simulink model "Posture_Regulation_NO_Singularity"  (R2022b)
settings: Solver=FixedStepAuto  StartTime=0.0  StopTime=10.0  MaxStep=0.1  RelTol=1e-3
values from neighbouring files (symbols this model uses):
  K = [3, 3, 1]    [AutomatedSimulation.m]
  theta_f = deg2rad(fc(3))    [AutomatedSimulation.m]
  theta_i = deg2rad(ans.output.signals.values(end,3))    [AutomatedSimulation.m]
  x_f = fc(1)    [AutomatedSimulation.m]
  x_i = ans.output.signals.values(end,1)    [AutomatedSimulation.m]
  y_f = fc(2)    [AutomatedSimulation.m]
  y_i = ans.output.signals.values(end,2)    [AutomatedSimulation.m]
libraries: simulink_extras x2
settings Model: Creator=Musta  LastModifiedBy=Musta

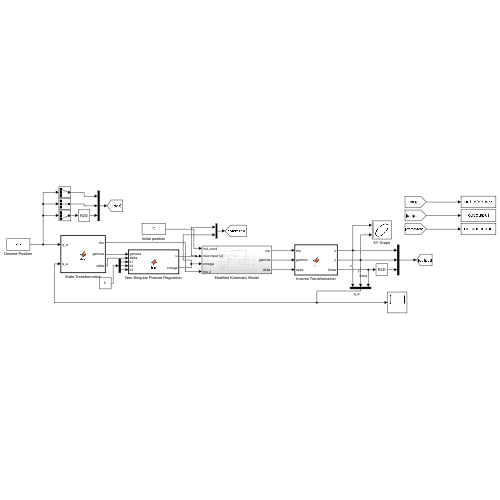
[thumbnail: Simulink's stored preview of the top-level diagram]
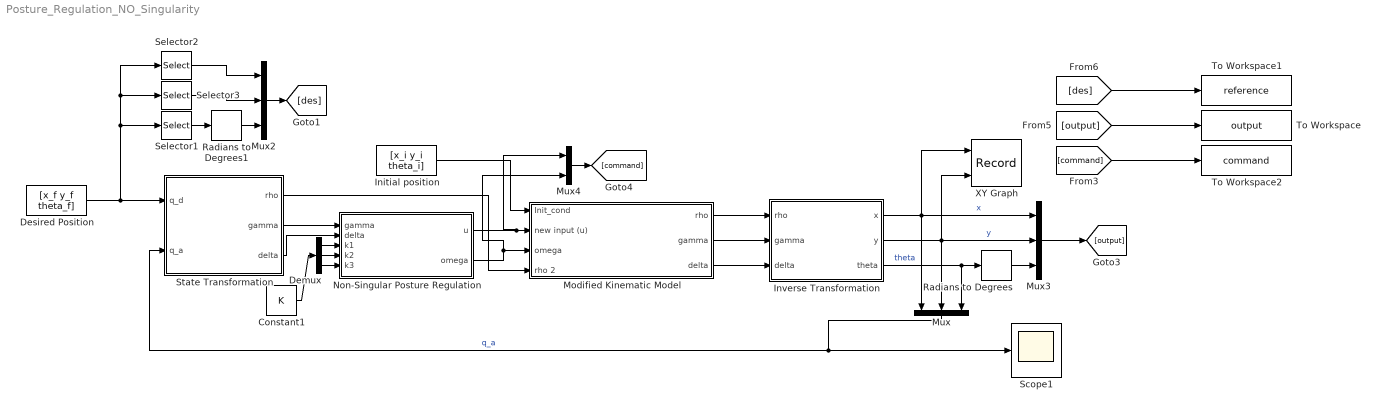
== system Posture_Regulation_NO_Singularity ==
  Constant1 : Constant  Value=K
  Demux : Demux  Outputs=3
  Desired Position : Constant  Value=[x_f y_f theta_f]
  Initial position : Constant  Value=[x_i y_i theta_i]
  Inverse Transformation : MATLAB Function  TreatAsAtomicUnit=on
  Modified Kinematic Model : Subsystem
  Mux : Mux  Inputs=3
  Mux2 : Mux  Inputs=3
  Mux3 : Mux  Inputs=3
  Mux4 : Mux  Inputs=2
  Non-Singular Posture Regulation : MATLAB Function  TreatAsAtomicUnit=on
  Radians to Degrees : simulink_extras/Transformations/Radians to Degrees
  Radians to Degrees1 : simulink_extras/Transformations/Radians to Degrees
  Scope1 : Scope
  Selector1 : Selector  InputPortWidth=3  IndexOptions=Index vector (dialog)  Indices=3  OutputSizes=1
  Selector2 : Selector  InputPortWidth=3  IndexOptions=Index vector (dialog)  Indices=1  OutputSizes=1
  Selector3 : Selector  InputPortWidth=3  IndexOptions=Index vector (dialog)  Indices=2  OutputSizes=1
  State Transformation : MATLAB Function  TreatAsAtomicUnit=on
  To Workspace : ToWorkspace  VariableName=output  SaveFormat=Structure With Time  SampleTime=-1
  To Workspace1 : ToWorkspace  VariableName=reference  SaveFormat=Structure With Time  SampleTime=-1
  To Workspace2 : ToWorkspace  VariableName=command  SaveFormat=Structure With Time  SampleTime=-1
  XY Graph : Record  FileSettingsInternal="{\"entries\":[{\"content\":{\"excelSettings\":{\"content\":{},\"type\":\"Streamout.ExcelSettings\"}},\"type\":\"Streamout.FileSettingStorage\",\"uuid\":\"c30e0c7c-8de7-4fd5-93f6-f23722b5ae44\"}],\"packageUris\":[\"http://schema.mathworks.com/mf0/streamout_blocks/R2020a\"],\"version\":\"1.0\"}"  Layout=[1 1]  SignalsInternal="{\"entries\":[{\"content\":{\"signals\":[{\"content\":{\"blockPath\":[\"Posture_Regulation_NO_Singularity/XY Graph\"],\"channel\":[],\"dimensions\":[1],\"domain\":\"Posture_Regulation_NO_Singularity/XY Graph\",\"lineColor\":\"#77ac30\",\"plots\":[],\"port\":1,\"sid\":[],\"signalID\":354,\"signalName\":\"x\"},\"type\":\"RecordBlkView.Signal\",\"uuid\":\"1f9c0edf-91b7-4929-98cb-a57c689434ed\"},{\"content\":{\"blockPath\":[\"Posture_Regulation_NO_Singularity/XY Graph\"],\"channel\":[],\"dimensions\":[1],\"domain\":\"Posture_Regulation_NO_Singularity/XY Graph\",\"lineColor\":\"#4dbeee\",\"plots\":[],\"port\":2,\"sid\":[],\"signalID\":357,\"signalName\":\"y\"},\"type\":\"RecordBlkView.Signal\",\"uuid\":\"3df65c5c-25b3-4ef8-84f3-e62cc3054bc7\"}]},\"type\":\"RecordBlkView.InputSignals\",\"uuid\":\"319c4578-7599-4632-be24-bc243958fcb7\"}],\"packageUris\":[\"http://schema.mathworks.com/mf0/streamout_blocks/R2020a\"],\"version\":\"1.0\"}"  VisualizationBindings="{\"xyplotplugin\":{\"info\":[{\"series\":[],\"subplotID\":1}]}}"  CompatibilityTag=XY
  wires:
  [command] -> To Workspace2/1
  [des] -> To Workspace1/1
  [output] -> To Workspace/1
  Selector2/1 -> Mux2/1
  Mux/1 -> Scope1/1, State Transformation/2(q_a)  "q_a"
  Selector3/1 -> Mux2/2
  Inverse Transformation/1(x) -> XY Graph/1, Mux/1, Mux3/1  "x"
  Desired Position/1 -> Selector2/1, Selector3/1, Selector1/1, State Transformation/1(q_d)
  Inverse Transformation/3(theta) -> Mux/3, Radians to Degrees/1  "theta"
  Radians to Degrees/1 -> Mux3/3
  Inverse Transformation/2(y) -> XY Graph/2, Mux3/2, Mux/2  "y"
  Modified Kinematic Model/3(delta) -> Inverse Transformation/3(delta)
  Mux2/1 -> [des]
  State Transformation/1(rho) -> Modified Kinematic Model/4(rho 2)
  Radians to Degrees1/1 -> Mux2/3
  Selector1/1 -> Radians to Degrees1/1
  Modified Kinematic Model/1(rho) -> Inverse Transformation/1(rho)
  Mux4/1 -> [command]
  State Transformation/2(gamma) -> Non-Singular Posture Regulation/1(gamma)
  Modified Kinematic Model/2(gamma) -> Inverse Transformation/2(gamma)
  State Transformation/3(delta) -> Non-Singular Posture Regulation/2(delta)
  Initial position/1 -> Modified Kinematic Model/1(Init_cond)
  Non-Singular Posture Regulation/1(u) -> Mux4/1, Modified Kinematic Model/2(new input (u))
  Mux3/1 -> [output]
  Non-Singular Posture Regulation/2(omega) -> Mux4/2, Modified Kinematic Model/3(omega)
  Constant1/1 -> Demux/1
  Demux/1 -> Non-Singular Posture Regulation/3(k1)
  Demux/2 -> Non-Singular Posture Regulation/4(k2)
  Demux/3 -> Non-Singular Posture Regulation/5(k3)

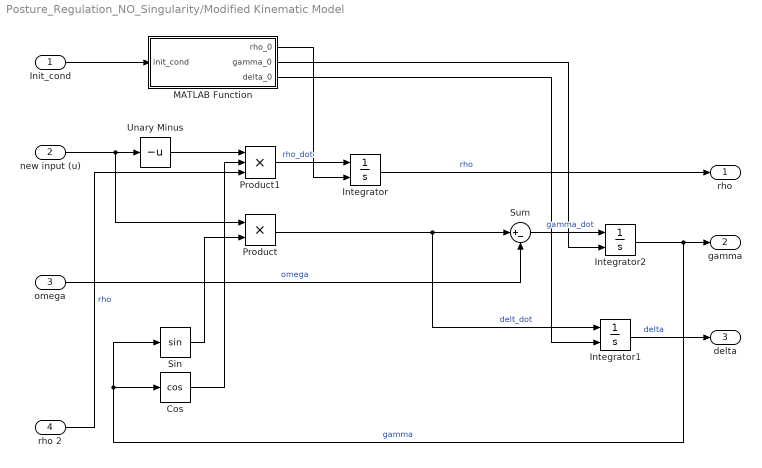
== system Posture_Regulation_NO_Singularity/Modified Kinematic Model ==
  Init_cond : Inport
  new input (u) : Inport  Port=2
  omega : Inport  Port=3
  rho 2 : Inport  Port=4
  Cos : Trigonometry  Operator=cos
  Integrator : Integrator  InitialConditionSource=external  InitialCondition=-10
  Integrator1 : Integrator  InitialConditionSource=external
  Integrator2 : Integrator  InitialConditionSource=external
  MATLAB Function : MATLAB Function  TreatAsAtomicUnit=on
  Product : Product
  Product1 : Product  Inputs=3
  Sin : Trigonometry
  Sum : Sum  Inputs=|+-
  Unary Minus : UnaryMinus
  rho : Outport
  gamma : Outport  Port=2
  delta : Outport  Port=3
  wires:
  Sum/1 -> Integrator2/1  "gamma_dot"
  Cos/1 -> Product1/2
  Unary Minus/1 -> Product1/1
  new input (u)/1 -> Product/1, Unary Minus/1
  Product1/1 -> Integrator/1  "rho_dot"
  Integrator/1 -> rho/1  "rho"
  Sin/1 -> Product/2
  Product/1 -> Sum/1, Integrator1/1  "delt_dot"
  omega/1 -> Sum/2  "omega"
  Integrator2/1 -> gamma/1, Cos/1, Sin/1  "gamma"
  Integrator1/1 -> delta/1  "delta"
  rho 2/1 -> Product1/3  "rho"
  Init_cond/1 -> MATLAB Function/1(init_cond)
  MATLAB Function/2(gamma_0) -> Integrator2/2
  MATLAB Function/3(delta_0) -> Integrator1/2
  MATLAB Function/1(rho_0) -> Integrator/2

== matlab function Posture_Regulation_NO_Singularity/Non-Singular Posture Regulation ==
  data: u output; omega output; gamma input; delta input; k1 input; k2 input; k3 input
function [u,omega] = fcn(gamma,delta, k1, k2, k3)

    u = k1 * cos(gamma);
    omega = k2 * gamma + (k1 * sin(gamma)*cos(gamma)/gamma * (gamma + k3 * delta));

end

== matlab function Posture_Regulation_NO_Singularity/State Transformation ==
  data: q_d input; rho output; q_a input; gamma output; delta output
function [rho,gamma,delta] = fcn(q_d, q_a)

    e_x = q_d(1) - q_a(1);
    e_y = q_d(2) - q_a(2);
    e_theta = q_d(3) - q_a(3);
    
    rho = sqrt(e_x^2 + e_y^2);
    gamma = mod(atan2(e_y,e_x),2*pi) - q_a(3);
    delta = gamma - e_theta;

end

== matlab function Posture_Regulation_NO_Singularity/Inverse Transformation ==
  data: x output; rho input; y output; gamma input; delta input; theta output
function [x,y,theta] = fcn(rho,gamma,delta)

    x = - rho * cos(delta);
    y = - rho * sin(delta);
    theta = delta - gamma;
    
end

== matlab function Posture_Regulation_NO_Singularity/Modified Kinematic Model/MATLAB Function ==
  data: init_cond input; rho_0 output; gamma_0 output; delta_0 output
function [rho_0, gamma_0, delta_0] = fcn(init_cond)

x_0 = init_cond(1);
y_0 = init_cond(2);
theta_0 = init_cond(3);


rho_0 = sqrt(x_0^2 + y_0^2);
gamma_0 = atan2(y_0,x_0) - theta_0 + pi;
delta_0 = gamma_0 + theta_0;
